simulink model "pd_controller"  (R2017a)
settings: Solver=ode4  StartTime=0.0  StopTime=5.0  FixedStep=1e-3  RelTol=1e-3
settings Model: Creator=Sean  LastModifiedBy=Sean

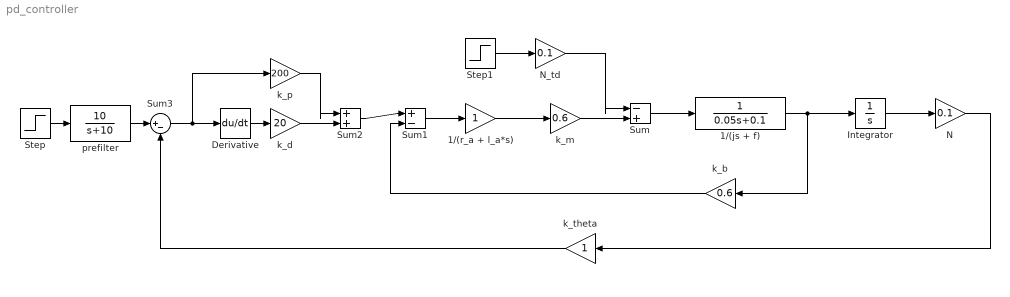
== system pd_controller ==
  1/(js + f) : TransferFcn  Denominator=[0.05 0.1]
  1/(r_a + l_a*s) : Gain
  Derivative : Derivative
  Integrator : Integrator
  N : Gain  Gain=0.1
  N_td : Gain  Gain=0.1
  Step : Step  SampleTime=0
  Step1 : Step  Time=3  After=120  SampleTime=0
  Sum : Sum  Inputs=|-+
  Sum1 : Sum  Inputs=|+-
  Sum2 : Sum  Inputs=|++
  Sum3 : Sum  Inputs=|+-
  k_b : Gain  Gain=0.6
  k_d : Gain  Gain=20
  k_m : Gain  Gain=0.6
  k_p : Gain  Gain=200
  k_theta : Gain
  prefilter : TransferFcn  Numerator=[10]  Denominator=[1 10]
  wires:
  1/(r_a + l_a*s)/1 -> k_m/1
  k_m/1 -> Sum/2
  Sum/1 -> 1/(js + f)/1
  1/(js + f)/1 -> k_b/1, Integrator/1
  Integrator/1 -> N/1
  Sum1/1 -> 1/(r_a + l_a*s)/1
  k_b/1 -> Sum1/2
  Sum2/1 -> Sum1/1
  k_d/1 -> Sum2/2
  k_p/1 -> Sum2/1
  Derivative/1 -> k_d/1
  Sum3/1 -> k_p/1, Derivative/1
  k_theta/1 -> Sum3/2
  N/1 -> k_theta/1
  Step1/1 -> N_td/1
  N_td/1 -> Sum/1
  Step/1 -> prefilter/1
  prefilter/1 -> Sum3/1
